simulink model "Testbench"  (R2025b)
settings: Solver=FixedStepDiscrete  StartTime=0.0  StopTime=size(bit_seq, 2) * 1E-3  FixedStep=1E-3  RelTol=1e-3
InitFcn:
  | bit_seq = [0 0 0 1 0 0 1 0 0 1];
libraries: dspswit3 x1
settings Model: Creator=abstract  LastModifiedBy=abstract
settings OptimizationCC: DefaultParameterBehavior=Inlined  EnhancedBackFolding=on  PassReuseOutputArgsAs=Individual arguments  ZeroExternalMemoryAtStartup=off  ZeroInternalMemoryAtStartup=off  OptimizeBlockOrder=speed  DifferentSizesBufferReuse=on  OptimizationCustomize=off  EfficientTunableParamExpr=on
settings DebuggingCC: ParameterTunabilityLossMsg=error
settings SFSimCC: MATLABDynamicMemAlloc=off
settings RTWCC: SystemTargetFile=ert.tlc  GenCodeOnly=on  TemplateMakefile=ert_default_tmf  Description=Embedded Coder
settings CodeAppCC: ForceParamTrailComments=on  IgnoreCustomStorageClasses=off  OperatorAnnotations=on  SimulinkDataObjDesc=on  SFDataObjDesc=on  InsertBlockDesc=on
settings ERTTargetCC: ERTCustomFileTemplate=example_file_process.tlc  TargetLangStandard=C99 (ISO)  GenerateSampleERTMain=on

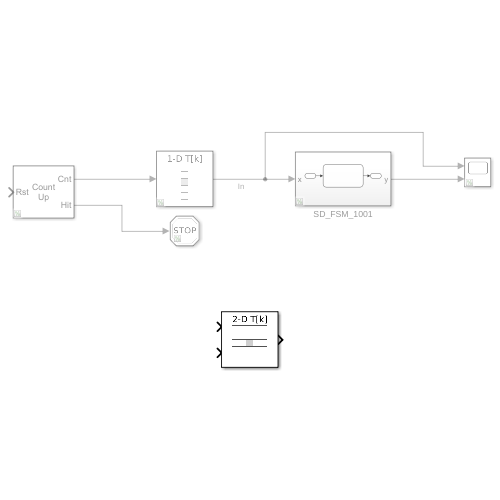
[thumbnail: Simulink's stored preview of the top-level diagram]
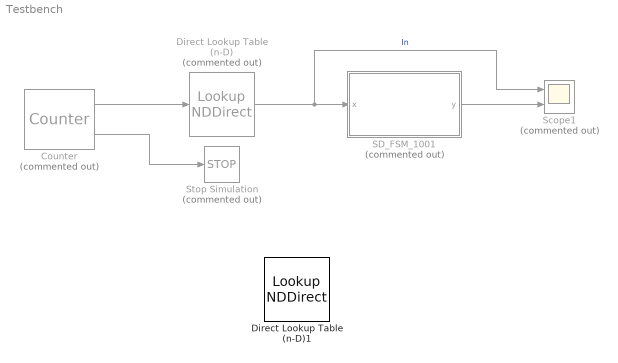
== system Testbench ==
  Counter : dspswit3/Counter  Commented=on  Direction=Up  CountEvent=Free running  CounterSize=User defined  MaxCount=size(bit_seq, 2) - 1  InitialCount=0  Output=Count and Hit  HitValue=size(bit_seq, 2) - 1  ResetInput=on  SamplesPerFrame=1  Ts=-1  CntDtype=uint8  HitDtype=Logical
  Direct Lookup Table (n-D) : LookupNDDirect  Commented=on  NumberOfTableDimensions=1  Table=bit_seq  TableDataTypeStr=fixdt(0,1,0)
  Direct Lookup Table (n-D)1 : LookupNDDirect
  SD_FSM_1001 : Subsystem  Commented=on
  Scope1 : Scope  Commented=on  NumInputPorts=2
      settings: ActiveDisplayYMinimum=-0.12499999999999997  ActiveDisplayYMaximum=1.125
  Stop Simulation : Stop  Commented=on
  wires:
  Counter/2 -> Stop Simulation/1
  Direct Lookup Table (n-D)/1 -> SD_FSM_1001/1(x), Scope1/1  "In"
  Counter/1 -> Direct Lookup Table (n-D)/1
  SD_FSM_1001/1(y) -> Scope1/2

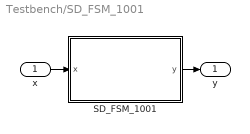
== system Testbench/SD_FSM_1001 ==
  x : Inport  OutDataTypeStr=fixdt(0,1,0)
  SD_FSM_1001 : Stateflow chart  TreatAsAtomicUnit=on
  y : Outport  OutDataTypeStr=fixdt(0,1,0)
  wires:
  x/1 -> SD_FSM_1001/1(x)
  SD_FSM_1001/1(y) -> y/1

== stateflow chart Testbench/SD_FSM_1001/SD_FSM_1001 ==
  settings: stateMachineType=MOORE_MACHINE  executeAtInitialization=1
  state S__
    y = 0;
  state S_1
    y = 0;
  state S_10
    y = 0;
  state S_100
    y = 0;
  state S_1001
    y = 1;
  S_100 -> S__ [order 2] : [x == 0]
  (default) -> S__
  S__ -> S__ [order 1] : [x == 0]
  S_1 -> S_1 [order 1] : [x == 1]
  S__ -> S_1 [order 2] : [x == 1]
  S_1 -> S_10 [order 2] : [x == 0]
  S_10 -> S_100 [order 1] : [x == 0]
  S_1001 -> S_1 [order 2] : [x == 1]
  S_10 -> S_1 [order 2] : [x == 1]
  S_1001 -> S_10 [order 1] : [x == 0]
  S_100 -> S_1001 [order 1] : [x == 1]
  data: x input fixdt(0,1,0); y output fixdt(0,1,0)
